simulink model "px4_bridge_udp"  (R2024b)
settings: Solver=VariableStepAuto  StartTime=0.0  StopTime=inf  RelTol=1e-3
model workspace (MAT data in the model file):
  NumVals = {4}
undefined symbols (not defined in the file): f
libraries: instrumentlib x2
settings Model: Creator=Nathan  LastModifiedBy=Nathan

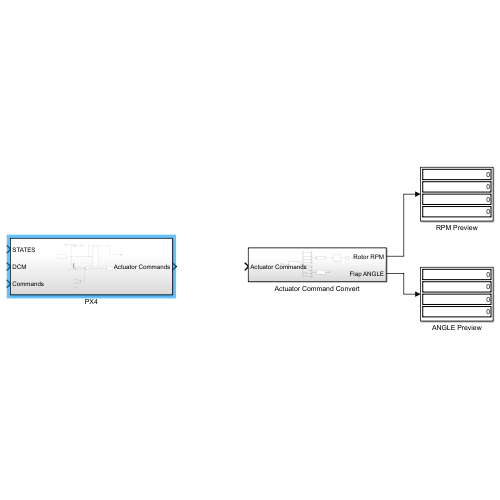
[thumbnail: Simulink's stored preview of the top-level diagram]
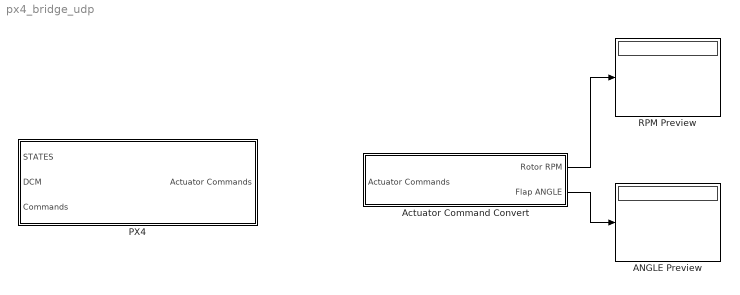
== system px4_bridge_udp ==
  ANGLE Preview : Display
  Actuator Command Convert : Subsystem
  PX4 : Subsystem
  RPM Preview : Display
  wires:
  Actuator Command Convert/1(Rotor RPM) -> RPM Preview/1
  Actuator Command Convert/2(Flap ANGLE) -> ANGLE Preview/1

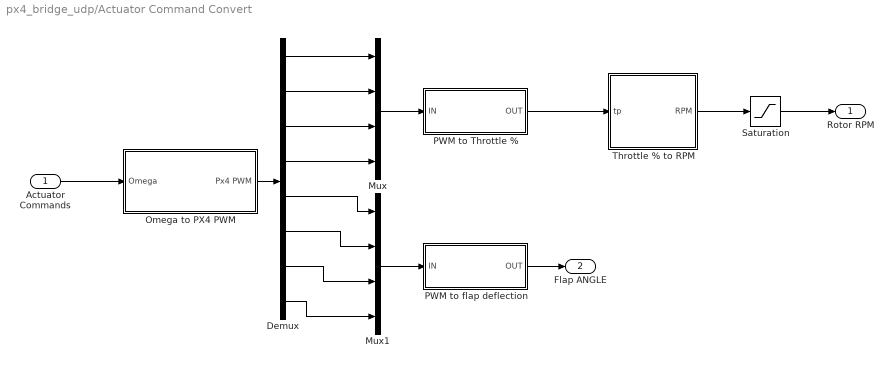
== system px4_bridge_udp/Actuator Command Convert ==
  Actuator Commands : Inport
  Demux : Demux  Outputs=8
  Mux : Mux
  Mux1 : Mux
  Omega to PX4 PWM : Subsystem
  PWM to Throttle % : Subsystem
  PWM to flap deflection : Subsystem
  Saturation : Saturate  UpperLimit=8000  LowerLimit=0
  Throttle % to RPM : MATLAB Function  TreatAsAtomicUnit=on
  Rotor RPM : Outport
  Flap ANGLE : Outport  Port=2
  wires:
  Actuator Commands/1 -> Omega to PX4 PWM/1(Omega)
  Omega to PX4 PWM/1(Px4 PWM) -> Demux/1
  Mux/1 -> PWM to Throttle %/1(IN)
  Demux/6 -> Mux1/2
  Demux/5 -> Mux1/1
  Mux1/1 -> PWM to flap deflection/1(IN)
  Demux/4 -> Mux/4
  Demux/3 -> Mux/3
  Demux/2 -> Mux/2
  Demux/1 -> Mux/1
  Demux/7 -> Mux1/3
  Demux/8 -> Mux1/4
  PWM to flap deflection/1(OUT) -> Flap ANGLE/1
  PWM to Throttle %/1(OUT) -> Throttle % to RPM/1(tp)
  Throttle % to RPM/1(RPM) -> Saturation/1
  Saturation/1 -> Rotor RPM/1

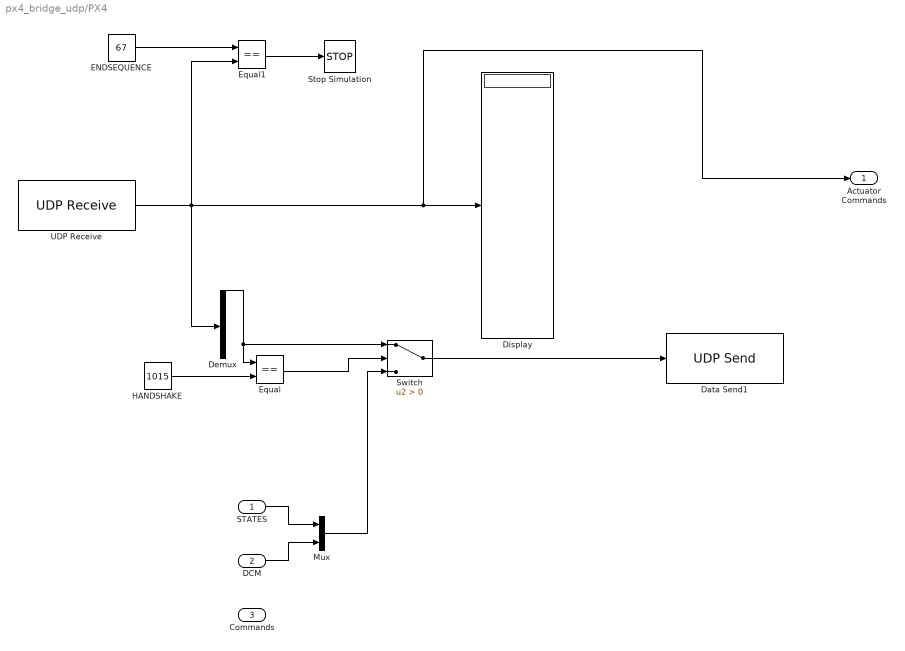
== system px4_bridge_udp/PX4 ==
  STATES : Inport
  DCM : Inport  Port=2
  Commands : Inport  Port=3
  Data Send1 : instrumentlib/UDP Send  Priority=1  Host=127.0.0.1  Port=65431  LocalAddress=0.0.0.0  LocalPort=-1  EnablePortSharing=off  OutputDatagramPacketSize=1024  ByteOrder=little-endian  EnableBlockingMode=on  SimulateUsing=Interpreted execution
  Demux : Demux  Outputs=16
  Display : Display
  ENDSEQUENCE : Constant  Value=67
  Equal : RelationalOperator  Operator===  OutDataTypeStr=boolean  RndMeth=Simplest  InputSameDT=off
  Equal1 : RelationalOperator  Operator===  OutDataTypeStr=boolean  RndMeth=Simplest  InputSameDT=off
  HANDSHAKE : Constant  Value=1015
  Mux : Mux  Inputs=2
  Stop Simulation : Stop
  Switch : Switch  Criteria=u2 > Threshold  SaturateOnIntegerOverflow=off  InputSameDT=off
  UDP Receive : instrumentlib/UDP Receive  Priority=2  LocalAddress=127.0.0.1  LocalPort=65432  EnablePortSharing=off  Host=localhost  Port=9090  GetLatestData=off  DataSize=[16]  DataType=double  ASCIIFormatting=%f,  Terminator=LF  CustomTerminator=10  ByteOrder=little-endian  EnableBlockingMode=on  Timeout=10  SampleTime=0.01  SimulateUsing=Interpreted execution
  Actuator Commands : Outport
  wires:
  UDP Receive/1 -> Actuator Commands/1, Display/1, Demux/1, Equal1/2
  HANDSHAKE/1 -> Equal/2
  Demux/1 -> Switch/1, Equal/1
  Equal/1 -> Switch/2
  Switch/1 -> Data Send1/1
  STATES/1 -> Mux/1
  DCM/1 -> Mux/2
  Mux/1 -> Switch/3
  Equal1/1 -> Stop Simulation/1
  ENDSEQUENCE/1 -> Equal1/1

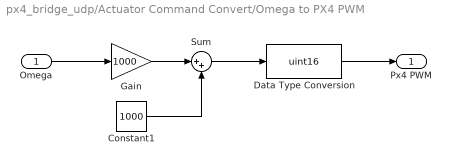
== system px4_bridge_udp/Actuator Command Convert/Omega to PX4 PWM ==
  Omega : Inport
  Constant1 : Constant  Value=1000
  Data Type Conversion : DataTypeConversion  OutDataTypeStr=uint16  SaturateOnIntegerOverflow=off  RndMeth=Floor
  Gain : Gain  Gain=1000
  Sum : Sum  Inputs=|++
  Px4 PWM : Outport
  wires:
  Data Type Conversion/1 -> Px4 PWM/1
  Sum/1 -> Data Type Conversion/1
  Omega/1 -> Gain/1
  Constant1/1 -> Sum/2
  Gain/1 -> Sum/1

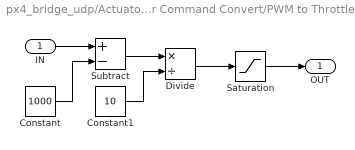
== system px4_bridge_udp/Actuator Command Convert/PWM to Throttle % ==
  IN : Inport
  Constant : Constant  Value=1000
  Constant1 : Constant  Value=10
  Divide : Product  Inputs=*/
  Saturation : Saturate  UpperLimit=100  LowerLimit=0
  Subtract : Sum  Inputs=+-
  OUT : Outport
  wires:
  Constant/1 -> Subtract/2
  IN/1 -> Subtract/1
  Divide/1 -> Saturation/1
  Subtract/1 -> Divide/1
  Saturation/1 -> OUT/1
  Constant1/1 -> Divide/2

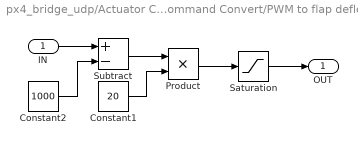
== system px4_bridge_udp/Actuator Command Convert/PWM to flap deflection ==
  IN : Inport
  Constant1 : Constant  Value=20
  Constant2 : Constant  Value=1000
  Product : Product
  Saturation : Saturate  UpperLimit=20  LowerLimit=-20
  Subtract : Sum  Inputs=+-
  OUT : Outport
  wires:
  IN/1 -> Subtract/1
  Constant2/1 -> Subtract/2
  Subtract/1 -> Product/1
  Product/1 -> Saturation/1
  Constant1/1 -> Product/2
  Saturation/1 -> OUT/1

== matlab function px4_bridge_udp/Actuator Command Convert/Throttle % to RPM ==
  data: tp input; RPM output
function RPM = fcn(tp)

RPM = zeros(size(tp));

for i = 1:numel(tp)
    RPM(i) = (27541.43 + (-0.08379553 - 27541.43)/(1 + (tp(i)/261.4585)^0.9851686));
end
